simulink model "DCMotor_Simple"  (R2016a)
settings: Solver=VariableStepAuto  StartTime=0.0  StopTime=5  RelTol=1e-3
settings Model: Creator=kkfrk  LastModifiedBy=kkfrk

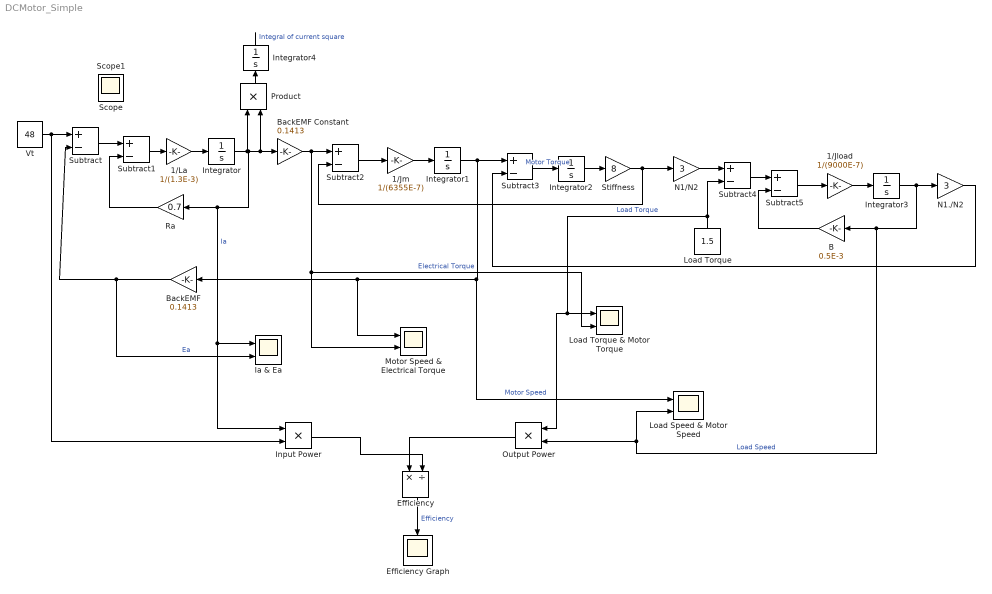
== system DCMotor_Simple ==
  1/Jload : Gain  Gain=1/(9000E-7)
  1/Jm : Gain  Gain=1/(6355E-7)
  1/La : Gain  Gain=1/(1.3E-3)
  B : Gain  Gain=0.5E-3
  BackEMF : Gain  Gain=0.1413
  BackEMF Constant : Gain  Gain=0.1413
  Efficiency : Product  Inputs=*/
  Efficiency Graph : Scope
  Ia & Ea : Scope  NumInputPorts=2
  Input Power : Product
  Integrator{,1..4} (5 alike) : Integrator
  Load Speed & Motor Speed : Scope  NumInputPorts=2
  Load Torque : Constant  Value=1.5
  Load Torque & Motor Torque : Scope  NumInputPorts=2
  Motor Speed & Electrical Torque : Scope  NumInputPorts=2
  N1./N2 : Gain  Gain=3
  N1/N2 : Gain  Gain=3
  Output Power : Product
  Product : Product
  Ra : Gain  Gain=0.7
  Stiffness : Gain  Gain=8
  Subtract{,1..5} (6 alike) : Sum  Inputs=+-
  Vt : Constant  Value=48
  Scope : Scope
  Scope1 : Scope
  wires:
  Vt/1 -> Input Power/2, Subtract/1
  Subtract/1 -> Subtract1/1
  Subtract1/1 -> 1/La/1
  1/La/1 -> Integrator/1
  Integrator/1 -> Product/2, BackEMF Constant/1, Ra/1, Ia & Ea/1, Input Power/1, Product/1  "Ia"
  Ra/1 -> Subtract1/2
  BackEMF Constant/1 -> Load Torque & Motor Torque/2, Motor Speed & Electrical Torque/2, Subtract2/1  "Electrical Torque"
  Subtract2/1 -> 1/Jm/1
  1/Jm/1 -> Integrator1/1
  Integrator1/1 -> Subtract3/1, Load Speed & Motor Speed/1, Motor Speed & Electrical Torque/1, BackEMF/1  "Motor Speed"
  BackEMF/1 -> Ia & Ea/2, Subtract/2  "Ea"
  Subtract3/1 -> Integrator2/1  "Motor Torque"
  Integrator2/1 -> Stiffness/1
  Stiffness/1 -> N1/N2/1, Subtract2/2
  N1/N2/1 -> Subtract4/1
  Load Torque/1 -> Load Torque & Motor Torque/1, Output Power/1, Subtract4/2  "Load Torque"
  Subtract4/1 -> Subtract5/1
  Subtract5/1 -> 1/Jload/1
  1/Jload/1 -> Integrator3/1
  Integrator3/1 -> Load Speed & Motor Speed/2, Output Power/2, B/1, N1./N2/1  "Load Speed"
  B/1 -> Subtract5/2
  N1./N2/1 -> Subtract3/2
  Output Power/1 -> Efficiency/1
  Input Power/1 -> Efficiency/2
  Efficiency/1 -> Efficiency Graph/1  "Efficiency"
  Product/1 -> Integrator4/1
  Integrator4/1 -> ?  "Integral of current square"
